simulink model "vehicle"  (R2020b)
settings: Solver=ode1be  StartTime=0.0  StopTime=10.0  FixedStep=ContIntTime  RelTol=1e-3
undefined symbols (not defined in the file): AmbTemp, batteryInternal_R_Ohm, batteryPackVoltage_V, GearRatio, hvBatterySOC_pct, motorDriveSimplePmsmDrv_rotorInertia_kg_m2, nominalCapacity_kWh
libraries: nesl_utility x10, fl_lib x9, ee_lib x2, sdl_lib x2
settings Model: DataDictionary=vehicle.sldd  Creator=Dmitry  LastModifiedBy=RomanHaziev

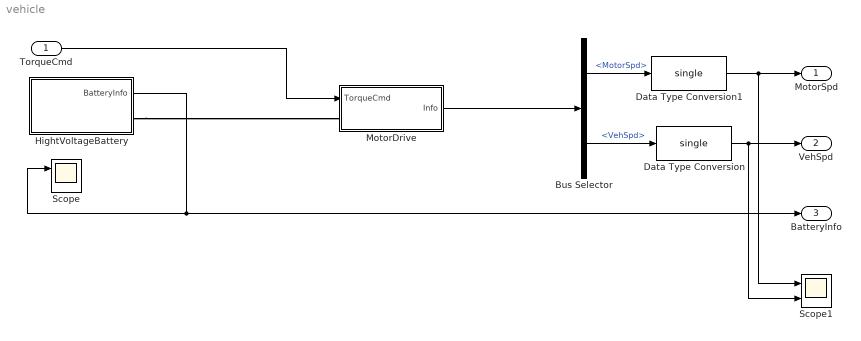
== system vehicle ==
  TorqueCmd : Inport  OutDataTypeStr=single
  Bus Selector : BusSelector  OutputSignals=MotorSpd,VehSpd
  Data Type Conversion : DataTypeConversion  OutDataTypeStr=single
  Data Type Conversion1 : DataTypeConversion  OutDataTypeStr=single
  HightVoltageBattery : Subsystem
  MotorDrive : Subsystem
  Scope : Scope  NumInputPorts=2
  Scope1 : Scope  NumInputPorts=2
  MotorSpd : Outport  OutDataTypeStr=single
  VehSpd : Outport  Port=2  OutDataTypeStr=single
  BatteryInfo : Outport  Port=3  OutDataTypeStr=Bus: BatteryInfo
  wires:
  TorqueCmd/1 -> MotorDrive/1(TorqueCmd)
  MotorDrive/1(Info) -> Bus Selector/1
  Bus Selector/2 -> Data Type Conversion/1  "<VehSpd>"
  Data Type Conversion/1 -> Scope1/2, VehSpd/1
  Bus Selector/1 -> Data Type Conversion1/1  "<MotorSpd>"
  HightVoltageBattery/1(BatteryInfo) -> Scope/1, BatteryInfo/1
  Data Type Conversion1/1 -> Scope1/1, MotorSpd/1
  connections:
  HightVoltageBattery/RConn1 -- MotorDrive/LConn1

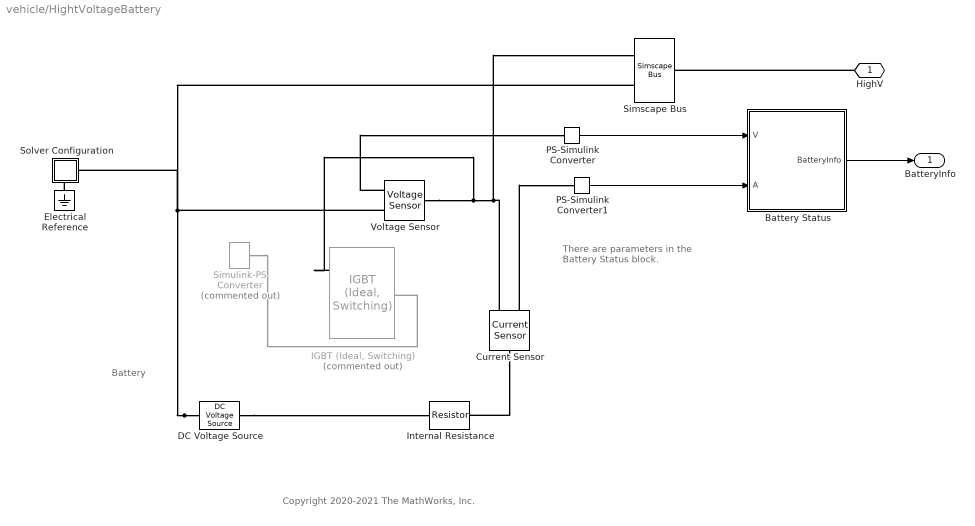
== system vehicle/HightVoltageBattery ==
  note: Battery
  note: There are parameters
      | in the Battery Status block.
  note: Copyright 2020-2021 The MathWorks, Inc.
  Battery Status : Subsystem
  Current Sensor : fl_lib/Electrical/Electrical Sensors/Current Sensor
  DC Voltage Source : fl_lib/Electrical/Electrical Sources/DC Voltage Source  v0=batteryPackVoltage_V V
      settings: AttributesFormatString=%<v0> [%<v0_unit>]
  Electrical Reference : fl_lib/Electrical/Electrical Elements/Electrical Reference
  "IGBT (Ideal, Switching)" : ee_lib/Semiconductors & Converters/IGBT (Ideal, Switching)  Commented=on  Vf=0.8 V  Ron=0.001 Ohm  Goff=1e-5 1/Ohm  Vth=6 V  diode_param=1  diode_Vf=0.8 V  diode_Ron=0.001 Ohm  diode_Goff=1e-5 1/Ohm  diode_C=50e-9 F  diode_iRM=-235 A  diode_iF=300 A  diode_idot=-50 A/us  diode_trr_param=1  diode_trr_factor=3  diode_trr=15 us  diode_Qrr=1500 s*uA  thermal_loss_option=ee.enum.converters.thermalLossOption.constantvalues  Von_data=[0, .1, .6, .8, 1, 1.3, 1.6, 2, 2.4; 0, .1, .7, 1, 1.2, 1.5, 1.9, 2.4, 2.8] V  Eon_data=[0, .0024, .024, .12, .2, .48, 1.04, 2.16, 3.24; 0, .003, .03, .15, .25, .6, 1.3, 2.7, 4.05] * 1e-3 J  Eoff_data=[0, .0007, .0066, .033, .066, .17, .33, .83, 1.5; 0, .001, .01, .05, .1, .25, .5, 1.2, 2.2] * 1e-3 J  Tj=[298.15, 398.15] K  Iout_data=[0, .1, 1, 5, 10, 20, 40, 70, 100] A  Eon_scalar=22.86e-3 J  Eoff_scalar=17.14e-3 J  Voff=300 V  Iout_scalar=600 A  diodeModelType=ee.enum.converters.diodeModelType.pwl  diode_IfMat=[.07, .12, .19, 1.75, 4.24, 7.32, 11.2; .16, .3, .72, 2.14, 4.02, 6.35, 9.12] A  diode_TjVec=[25, 125] degC  diode_VfVec=[.5, .7, .9, 1.3, 1.7, 2.1, 2.5] V  thermal_network_parameterization=ee.enum.thermalNetworkTopology.external  Rth=[.08, .5] K/W  Rth_Foster=[.08, .14, .22, .16] K/W  thermal_mass_parameterization=ee.enum.thermalNetwork.timeconstant  thermal_mass=[.01, .5] J/K  thermal_mass_Foster=[.001, .005, .05, .5] J/K  thermal_time_constant=[.001, .2] s  thermal_time_constant_Foster=[7e-05, .0007, .01, .08] s  thermal_mass_initial_temperatures=[25, 25] degC  junction_thermal_mass=0.01 J/K  Tau=1e-4 s  vT_specify=off  vT_priority=None  vT=0 V  vT_nominal_specify=off  vT_nominal_unit=V  vT_nominal_value=1  Qj_specify=off  Qj_priority=None  Qj=0 W  Qj_nominal_specify=off  Qj_nominal_unit=W  Qj_nominal_value=1  junction_temperature_specify=off  junction_temperature_priority=None  junction_temperature=25 degC  junction_temperature_nominal_specify=off  junction_temperature_nominal_unit=degC  junction_temperature_nominal_value=1
  Internal Resistance : fl_lib/Electrical/Electrical Elements/Resistor  R=batteryInternal_R_Ohm Ohm  i_specify=off  i_priority=High  i=0 A  i_nominal_specify=off  i_nominal_unit=A  i_nominal_value=1  v_specify=off  v_priority=High  v=0 V  v_nominal_specify=off  v_nominal_unit=V  v_nominal_value=1
      settings: AttributesFormatString=%<R> [%<R_unit>]
  PS-Simulink Converter : nesl_utility/PS-Simulink Converter  PhysicalDomain=network_engine_domain  SubClassName=ps_output  LeftPortType=input  RightPortType=output  PseudoPeriodic=off  Frequencies=[]  Unit=inherit  AffineConversion=off
  PS-Simulink Converter1 : nesl_utility/PS-Simulink Converter  PhysicalDomain=network_engine_domain  SubClassName=ps_output  LeftPortType=input  RightPortType=output  PseudoPeriodic=off  Frequencies=[]  Unit=inherit  AffineConversion=off
  Simscape Bus : SimscapeBus  HierarchyStrings=plus;minus
  Simulink-PS Converter : nesl_utility/Simulink-PS Converter  Commented=on  PhysicalDomain=network_engine_domain  SubClassName=ps_input  LeftPortType=input  RightPortType=output  PseudoPeriodic=off  Frequencies=[]  NoiseDistribution=none  NoiseParameters=[]  Unit=V  AffineConversion=off  FilteringAndDerivatives=zero  SimscapeFilterOrder=1  InputFilterTimeConstant=.001  UdotUserProvided=0
  Solver Configuration : Subsystem
      settings: PortSchema="{\"entries\":[{\"content\":{\"sides\":[{\"content\":{\"connectorIds\":[]},\"type\":\"ConnectorPlacement.EquallySpacedRectSide\",\"uuid\":\"4a7e26c2-e9e9-4fea-b605-533b1a682be7\"},{\"content\":{\"connectorIds\":[\"RConn1\"],\"side\":\"RIGHT\"},\"type\":\"ConnectorPlacement.EquallySpacedRectSide\",\"uuid\":\"0210e324-555e-4372-b836-fcc8ab23e933\"},{\"content\":{\"connectorIds\":[],\"side\":\"TOP\"},\"type\":\"ConnectorPlacement.EquallySpacedRectSide\",\"uuid\":\"9bbae011-e6fc-4534-a44f-d79a5697c939\"},{\"content\":{\"connectorIds\":[\"RConn2\"],\"side\":\"BOTTOM\"},\"type\":\"ConnectorPlacement.EquallySpacedRectSide\",\"uuid\":\"d5829c0a-26ea-402d-a1c6-900997ddf1a8\"}]},\"type\":\"ConnectorPlacement.EquallySpacedConnector\",\"uuid\":\"f4e17c65-54c6-42fe-a467-9c6b014b697a\"}],\"packageUris\":[\"http://schema.mathworks.com/mf0/Connector/19700101\"],\"version\":\"1.0\"}"
  Voltage Sensor : fl_lib/Electrical/Electrical Sensors/Voltage Sensor
  HighV : PMIOPort  Side=Right
  BatteryInfo : Outport  OutDataTypeStr=Bus: BatteryInfo
  wires:
  PS-Simulink Converter1/1 -> Battery Status/2(A)
  Battery Status/1(BatteryInfo) -> BatteryInfo/1
  PS-Simulink Converter/1 -> Battery Status/1(V)
  connections:
  Current Sensor/LConn1 -- Internal Resistance/RConn1
  DC Voltage Source/LConn1 -- Internal Resistance/LConn1
  HighV/RConn1 -- Simscape Bus/RConn1
  Voltage Sensor/RConn1 -- PS-Simulink Converter/LConn1
  Current Sensor/RConn1 -- PS-Simulink Converter1/LConn1
  Electrical Reference/LConn1 -- Solver Configuration/RConn2
  DC Voltage Source/RConn1 -- Simscape Bus/LConn2 -- Solver Configuration/RConn1 -- Voltage Sensor/RConn2
  Voltage Sensor/LConn1 -- "IGBT (Ideal, Switching)"/RConn2 -- Current Sensor/RConn2 -- Simscape Bus/LConn1
  Simulink-PS Converter/RConn1 -- "IGBT (Ideal, Switching)"/LConn1

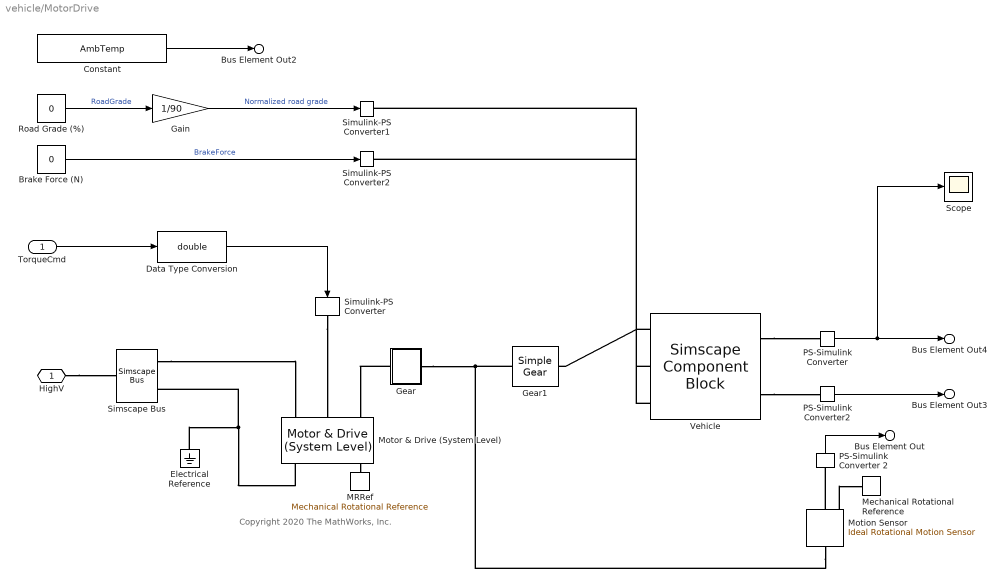
== system vehicle/MotorDrive ==
  note: Copyright 2020 The MathWorks, Inc.
  TorqueCmd : Inport  OutDataTypeStr=single  Unit=N*m
      settings: AttributesFormatString=%<Unit>
  " Simscape Bus" : SimscapeBus  HierarchyStrings=plus;minus
  Brake Force (N) : Constant  Value=0
  Constant : Constant  Value=AmbTemp
  Data Type Conversion : DataTypeConversion  OutDataTypeStr=double
  Electrical Reference : fl_lib/Electrical/Electrical Elements/Electrical Reference
  Gain : Gain  Gain=1/90
  Gear : Subsystem
  Gear1 : sdl_lib/Gears/Simple Gear  ratio=GearRatio  rotation_direction=sdl.enum.shaftOutputDirection.same  friction_model=sdl.enum.gear_efficiencies_load.constant  mu_visc=[0, 0] N*m/(rad/s)  T_noload=0.1 N*m  T_nom=5 N*m  efficiency_nom=0.9  efficiency=GearEfficiency  temperature_TLU=[280, 300, 320] K  load_TLU=[1, 5, 10] N*m  efficiency_TLU=[.95, .9, .85]  efficiency_TLU2=[.85, .8, .75; .95, .9, .85; .85, .8, .7]  w_thr=0.01 rad/s  pwr_thr=0.001 W  thermal_mass=50 J/K  enable_faults=simscape.enum.onoff.off  efficiency_fault=0.05  external_fault=simscape.enum.onoff.off  temporal_fault=simscape.enum.onoff.off  fault_time=5 s  fault_angles=pi / 12 rad  report_fault=simscape.enum.assert.action.none  temperature_specify=off  temperature_priority=High  temperature=300 K  temperature_nominal_specify=off  temperature_nominal_unit=K  temperature_nominal_value=1
      settings: AttributesFormatString=%<ratio>
  MRRef : fl_lib/Mechanical/Rotational Elements/Mechanical Rotational Reference
  Mechanical Rotational Reference : fl_lib/Mechanical/Rotational Elements/Mechanical Rotational Reference
  Motion Sensor : fl_lib/Mechanical/Mechanical Sensors/Ideal Rotational Motion Sensor  wrap_angle=simscape.enum.onoff.off  offset=0 rad
  Motor & Drive (System Level) : ee_lib/Electromechanical/Motor & Drive (System Level)  torque_speed_param=ee.enum.electromech.envelope.torque_power  overtorque_param=ee.enum.electromech.overtorque.no  T_t=[.09, .08, .07, 0] N*m  T_t_intermittent=[.36, .32, .28, 0] N*m  w_t=[0, 3750, 7500, 8000] rpm  torque_max=motorDriveSimplePmsmDrv_trqMax_Nm N*m  power_max=motorDriveSimplePmsmDrv_powMax_W W  torque_max_intermittent=0.4 N*m  power_max_intermittent=120 W  time_overtorque=30 s  time_recover=60 s  Tc=motorDriveSimplePmsmDrv_timeConst_s s  losses_param=2  eff=100  w_eff=3750 rpm  T_eff=0.08 N*m  Piron=0 W  Pbase=0 W  w_eff_vec=motorDriveSimplePmsmDrv_spdVec_rpm rpm  T_eff_vec=motorDriveSimplePmsmDrv_trqVec_Nm N*m  v_eff_vec=[100, 250, 400] V  losses_mat=motorDriveSimplePmsmDrv_LossTbl_W W  efficiency_mat=[95, 95, 95, 95; 95, 95, 95, 95; 95, 95, 95, 95; 95, 95, 95, 95; 95, 95, 95, 95]  losses_mat_3D=ones(5, 4, 3) W  efficiency_mat_3D=95 * ones(5, 4, 3)  Res=0 Ohm  J=motorDriveSimplePmsmDrv_rotorInertia_kg_m2 kg*m^2  lam=motorDriveSimplePmsmDrv_rotorDamping_Nm_per_radps N*m/(rad/s)  speed0=motorDriveSimplePmsmDrv_initialRotorSpd_rpm rpm  faulted_specify=off  faulted_priority=None  faulted=0  faulted_nominal_specify=off  faulted_nominal_unit=1  faulted_nominal_value=1  torqueLimitContinuous_specify=off  torqueLimitContinuous_priority=None  torqueLimitContinuous=0 N*m  torqueLimitContinuous_nominal_specify=off  torqueLimitContinuous_nominal_unit=N*m  torqueLimitContinuous_nominal_value=1  alpha=3.93e-3 1/K  Tmeas=25 degC  Tmeas2=125 degC  losses_mat_T2=[1.49, 1.74, 2.49, 3.74; .42, .67, 1.42, 2.67; .06, .31, 1.06, 2.31; .42, .67, 1.42, 2.67; 1.49, 1.74, 2.49, 3.74] W  efficiency_mat_T2=[95, 95, 95, 95; 95, 95, 95, 95; 95, 95, 95, 95; 95, 95, 95, 95; 95, 95, 95, 95]  losses_mat_3D_T2=ones(5, 4, 3) W  efficiency_mat_3D_T2=95 * ones(5, 4, 3)  thermal_mass=100 J/K  initial_temperature=25 degC  fault_condition=1  fault_threshold=0.5
      settings: SourceProductBaseCode=PS  LogSimulationData=on
  PS-Simulink Converter : nesl_utility/PS-Simulink Converter  PhysicalDomain=network_engine_domain  SubClassName=ps_output  LeftPortType=input  RightPortType=output  PseudoPeriodic=off  Frequencies=[]  Unit=km/hr  AffineConversion=off
  PS-Simulink Converter 2 : nesl_utility/PS-Simulink Converter  PhysicalDomain=network_engine_domain  SubClassName=ps_output  LeftPortType=input  RightPortType=output  PseudoPeriodic=off  Frequencies=[]  Unit=rpm  AffineConversion=off
  PS-Simulink Converter2 : nesl_utility/PS-Simulink Converter  PhysicalDomain=network_engine_domain  SubClassName=ps_output  LeftPortType=input  RightPortType=output  PseudoPeriodic=off  Frequencies=[]  Unit=1  AffineConversion=off
  Road Grade (%) : Constant  Value=0
  Scope : Scope
  Simulink-PS Converter : nesl_utility/Simulink-PS Converter  PhysicalDomain=network_engine_domain  SubClassName=ps_input  LeftPortType=input  RightPortType=output  PseudoPeriodic=off  Frequencies=[]  NoiseDistribution=none  NoiseParameters=[]  Unit=N*m  AffineConversion=off  FilteringAndDerivatives=zero  SimscapeFilterOrder=1  InputFilterTimeConstant=.001  UdotUserProvided=0
  Simulink-PS Converter1 : nesl_utility/Simulink-PS Converter  PhysicalDomain=network_engine_domain  SubClassName=ps_input  LeftPortType=input  RightPortType=output  PseudoPeriodic=off  Frequencies=[]  NoiseDistribution=none  NoiseParameters=[]  Unit=1  AffineConversion=off  FilteringAndDerivatives=provide  SimscapeFilterOrder=1  InputFilterTimeConstant=0.001  UdotUserProvided=0
  Simulink-PS Converter2 : nesl_utility/Simulink-PS Converter  PhysicalDomain=network_engine_domain  SubClassName=ps_input  LeftPortType=input  RightPortType=output  PseudoPeriodic=off  Frequencies=[]  NoiseDistribution=none  NoiseParameters=[]  Unit=N  AffineConversion=off  FilteringAndDerivatives=provide  SimscapeFilterOrder=1  InputFilterTimeConstant=0.001  UdotUserProvided=0
  Vehicle : SimscapeComponentBlock  SourceFile=Vehicle1DBasic  ComponentPath=Vehicle1DBasic  ComponentVariants="[\"Vehicle1DBasic\"]"  ComponentVariantNames="[\"Vehicle1DBasic\"]"  ClassName=Vehicle1DBasic  SchemaVersion=1  M_e=vehicleVehMass_kg kg  R_tire=vehicleTireRollingRadius_cm cm  A_rl=vehicleRoadLoadA_N N  B_rl=vehicleRoadLoadB_N_per_kph N*hr/km  C_rl=vehicleRoadLoadB_N_per_kph2 N*hr^2/km^2  ShowBrakeIn=simscape.enum.onoff.on  ShowGradeIn=simscape.enum.onoff.on  grav=9.81 m/s^2  ShowVelOut=simscape.enum.onoff.on  ShowGOut=simscape.enum.onoff.on  v_specify=off  v_priority=High  v=0 km/hr  v_nominal_specify=off  v_nominal_unit=km/hr  v_nominal_value=1
      settings: CopyFcn=simscape.engine.sli.internal.componentblockcallback(gcbh,'COPY')  PreCopyFcn=simscape.engine.sli.internal.componentblockcallback(gcbh,'PRECOPY')  PreDeleteFcn=simscape.engine.sli.internal.componentblockcallback(gcbh,'PREDELETE')  InternalSimscapePortConfiguration="{\"Bottom\":[],\"Left\":[{\"id\":\"Axle\",\"label\":\"Axle\",\"type\":\"foundation.mechanical.rotational.rotational\"}],\"Right\":[{\"id\":\"v_out\",\"label\":\"V\",\"type\":\"output\"},{\"id\":\"G\",\"label\":\"G\",\"type\":\"output\"}],\"Top\":[{\"id\":\"brkF\",\"label\":\"Brake\",\"type\":\"input\"},{\"id\":\"grade_norm\",\"label\":\"Grade\",\"type\":\"input\"}]}"
      mask Type: Vehicle 1D Basic
  HighV : PMIOPort  Side=Left
  Bus Element Out : Outport  PortName=Info  Element=MotorSpd
      settings: AttributesFormatString=%<Unit>
  Bus Element Out2 : Outport  PortName=Info  Element=Temp
      settings: AttributesFormatString=%<Unit>
  Bus Element Out3 : Outport  PortName=Info  Element=G
      settings: AttributesFormatString=%<Unit>
  Bus Element Out4 : Outport  PortName=Info  Element=VehSpd
      settings: AttributesFormatString=%<Unit>
  wires:
  PS-Simulink Converter 2/1 -> Bus Element Out/1
  Constant/1 -> Bus Element Out2/1
  Gain/1 -> Simulink-PS Converter1/1  "Normalized road grade"
  PS-Simulink Converter2/1 -> Bus Element Out3/1
  PS-Simulink Converter/1 -> Scope/1, Bus Element Out4/1
  Road Grade (%)/1 -> Gain/1  "RoadGrade"
  Brake Force (N)/1 -> Simulink-PS Converter2/1  "BrakeForce"
  TorqueCmd/1 -> Data Type Conversion/1
  Data Type Conversion/1 -> Simulink-PS Converter/1
  connections:
  Motor & Drive (System Level)/RConn1 -- " Simscape Bus"/LConn2 -- Electrical Reference/LConn1
  Motion Sensor/LConn1 -- Gear1/LConn1 -- Gear/RConn1
  Gear/LConn1 -- Motor & Drive (System Level)/LConn3
  Motion Sensor/RConn2 -- PS-Simulink Converter 2/LConn1
  HighV/RConn1 -- " Simscape Bus"/RConn1
  Motion Sensor/RConn1 -- Mechanical Rotational Reference/LConn1
  Motor & Drive (System Level)/RConn3 -- MRRef/LConn1
  Simulink-PS Converter/RConn1 -- Motor & Drive (System Level)/LConn2
  Vehicle/LConn1 -- Gear1/RConn1
  Vehicle/RConn1 -- PS-Simulink Converter/LConn1
  Vehicle/RConn2 -- PS-Simulink Converter2/LConn1
  Vehicle/LConn2 -- Simulink-PS Converter2/RConn1
  Vehicle/LConn3 -- Simulink-PS Converter1/RConn1
  " Simscape Bus"/LConn1 -- Motor & Drive (System Level)/LConn1

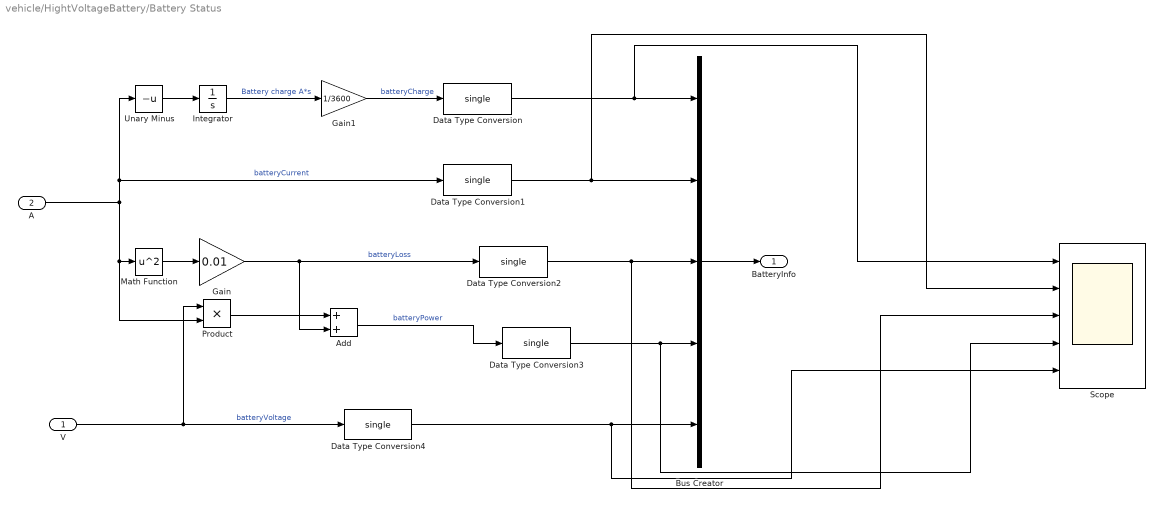
== system vehicle/HightVoltageBattery/Battery Status ==
  V : Inport
  A : Inport  Port=2
  Add : Sum
  Bus Creator : BusCreator  Inputs=5  OutDataTypeStr=Bus: BatteryInfo
      settings: InheritFromInputs=off
  Data Type Conversion{,1..4} (5 alike) : DataTypeConversion  OutDataTypeStr=single
  Gain : Gain  Gain=0.01
  Gain1 : Gain  Gain=1/3600
  Integrator : Integrator  InitialCondition=nominalCapacity_kWh/batteryPackVoltage_V*1000*hvBatterySOC_pct/100*3600
  Math Function : Math  Operator=square  SaturateOnIntegerOverflow=on
  Product : Product
  Scope : Scope  NumInputPorts=5
  Unary Minus : UnaryMinus
  BatteryInfo : Outport  OutDataTypeStr=Bus: BatteryInfo
  wires:
  Gain1/1 -> Data Type Conversion/1  "batteryCharge"
  Unary Minus/1 -> Integrator/1
  Gain/1 -> Add/2, Data Type Conversion2/1  "batteryLoss"
  Product/1 -> Add/1
  Integrator/1 -> Gain1/1  "Battery charge A*s"
  Add/1 -> Data Type Conversion3/1  "batteryPower"
  Math Function/1 -> Gain/1
  Bus Creator/1 -> BatteryInfo/1
  A/1 -> Data Type Conversion1/1, Unary Minus/1, Math Function/1, Product/2  "batteryCurrent"
  V/1 -> Data Type Conversion4/1, Product/1  "batteryVoltage"
  Data Type Conversion/1 -> Scope/1, Bus Creator/1
  Data Type Conversion1/1 -> Scope/2, Bus Creator/2
  Data Type Conversion2/1 -> Scope/3, Bus Creator/3
  Data Type Conversion3/1 -> Scope/4, Bus Creator/4
  Data Type Conversion4/1 -> Scope/5, Bus Creator/5

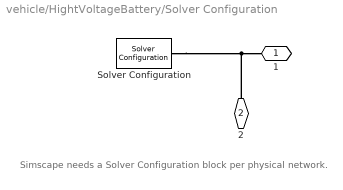
== system vehicle/HightVoltageBattery/Solver Configuration ==
  note: Simscape needs a Solver Configuration block per physical network.
  Solver Configuration : nesl_utility/Solver Configuration  PhysicalDomain=network_engine_domain  SubClassName=solver  LeftPortType=input  RightPortType=generic  Tones=[]  Harmonics=[]  SimulateNoise=off  Profile=off  UseLocalSampling=off  EnableSwitchedLinearOptims=on  FrequencyDomain=off  UseCCode=off  RelTol=0.001  AbsTol=1e-06  MinStep=1e-09  ToWorkspace=off  RevertToSquareIcSolve=off  NumHomotopyIterations=100  PhasorMode=off  PhasorModeNumHarmonics=1  DoDC=off  ResidualTolerance=1e-6  UseLocalSolver=off  LocalSolverChoice=NE_BACKWARD_EULER_ADVANCER  LocalSolverSampleTime=0.01  DoFixedCost=off  MaxNonlinIter=3  MaxModeIter=2  ComputeImpulses=off  ImpulseIterations=2  LinearAlgebra=auto  EquationFormulation=NE_TIME_EF  DelaysMemoryBudget=1024  AutomaticFiltering=on  FilteringTimeConstant=ContIntTime  PartitionStorageMethod=AS_NEEDED  PartitionMemoryBudget=1024  PartitionMethod=FAST
      settings: AttributesFormatString=Local solver %<UseLocalSolver>
  1 : PMIOPort  Side=Right
  2 : PMIOPort  Port=2  Side=Right
  connections:
  Solver Configuration/RConn1 -- 1/RConn1 -- 2/RConn1

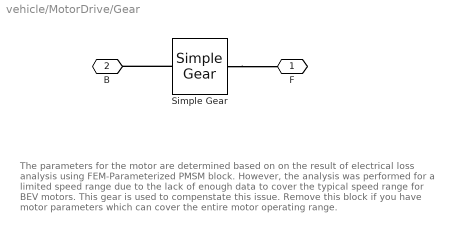
== system vehicle/MotorDrive/Gear ==
  note: The parameters for the motor are determined based on on the result of electrical loss analysis using FEM-Parameterized PMSM block. However, the analysis was performed for a limited speed range due to the lack of enough data to cover the typical speed range for BEV motors. This gear is used to compenstate this issue. Remove this block if you have motor parameters which can cover the entire motor operating range.
  Simple Gear : sdl_lib/Gears/Simple Gear  ratio=double(3/GearRatio)  rotation_direction=sdl.enum.shaftOutputDirection.same  friction_model=sdl.enum.gear_efficiencies_load.off  mu_visc=[0, 0] N*m/(rad/s)  T_noload=0.1 N*m  T_nom=5 N*m  efficiency_nom=0.8  efficiency=0.8  temperature_TLU=[280, 300, 320] K  load_TLU=[1, 5, 10] N*m  efficiency_TLU=[.95, .9, .85]  efficiency_TLU2=[.85, .8, .75; .95, .9, .85; .85, .8, .7]  w_thr=0.01 rad/s  pwr_thr=0.001 W  thermal_mass=50 J/K  enable_faults=simscape.enum.onoff.off  efficiency_fault=0.05  external_fault=simscape.enum.onoff.off  temporal_fault=simscape.enum.onoff.off  fault_time=5 s  fault_angles=pi / 12 rad  report_fault=simscape.enum.assert.action.none  temperature_specify=off  temperature_priority=High  temperature=300 K  temperature_nominal_specify=off  temperature_nominal_unit=K  temperature_nominal_value=1
      settings: AttributesFormatString=%<ratio>
  F : PMIOPort  Side=Right
  B : PMIOPort  Port=2  Side=Left
  connections:
  Simple Gear/RConn1 -- F/RConn1
  Simple Gear/LConn1 -- B/RConn1
